simulink model "voltage_to_kelvin_testing"  (R2015a)
settings: Solver=ode45  StartTime=0.0  StopTime=10.0  RelTol=1e-3
libraries: simulink x1
settings Model: Creator=USER  LastModifiedBy=USER

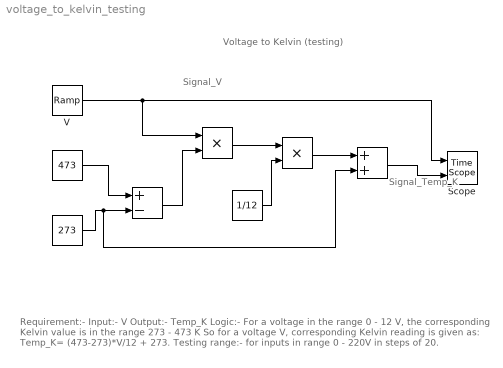
== system voltage_to_kelvin_testing ==
  note: Signal_V
  note: Signal_Temp_K
  note: Requirement:-
      |
      | Input:- V
      | Output:- Temp_K
      | Logic:- For a voltage in the range 0 - 12 V, the corresponding Kelvin value is in the range 273 - 473 K
      | 	     So for a voltage V, corresponding Kelvin reading is given as:
      | 	     Temp_K= (473-273)*V/12 + 273.
      | Testing range:- for inputs in range 0 - 220V in steps of 20.
  note: Voltage to Kelvin (testing)
  " " : Constant  Value=473
  "  " : Constant  Value=273
  "   " : Constant  Value=1/12
  "    " : Product
  "     " : Sum  Inputs=+-
  "      " : Sum
  "       " : Product
  Scope : TimeScope  NumInputPorts=2
  V : simulink/Sources/Ramp  slope=11  start=0  X0=0
  wires:
  " "/1 -> "     "/1
  "  "/1 -> "      "/2, "     "/2
  V/1 -> Scope/1, "    "/1
  "     "/1 -> "    "/2
  "    "/1 -> "       "/1
  "   "/1 -> "       "/2
  "       "/1 -> "      "/1
  "      "/1 -> Scope/2
